simulink model "Dinamica_Residual"  (R2023b)
settings: Solver=VariableStepAuto  StartTime=0.0  StopTime=10.0  RelTol=1e-3
values from neighbouring files (symbols this model uses):
  lambda_m = 0.016    [parametros_proyecto2.m]
  Ld = 6.6e-3    (= 0.0066)    [parametros_proyecto2.m]
  Lls = 0.8e-3    (= 0.0008)    [parametros_proyecto2.m]
  Lq = 5.8e-3    (= 0.0058)    [parametros_proyecto2.m]
  r = 120    [parametros_proyecto2.m]
  Rs_ref = 1.02    [parametros_proyecto2.m]
  Rts_amb = 146.7    [parametros_proyecto2.m]
undefined symbols (not defined in the file or in its folder): b_eq, cts, J_eq, P_p, R_s
settings Model: Creator=ignab  LastModifiedBy=ignab

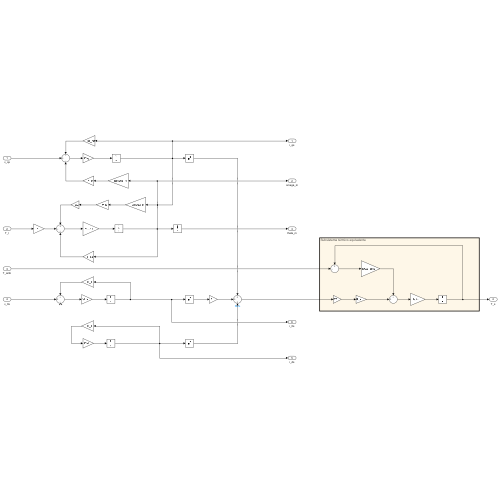
[thumbnail: Simulink's stored preview of the top-level diagram]
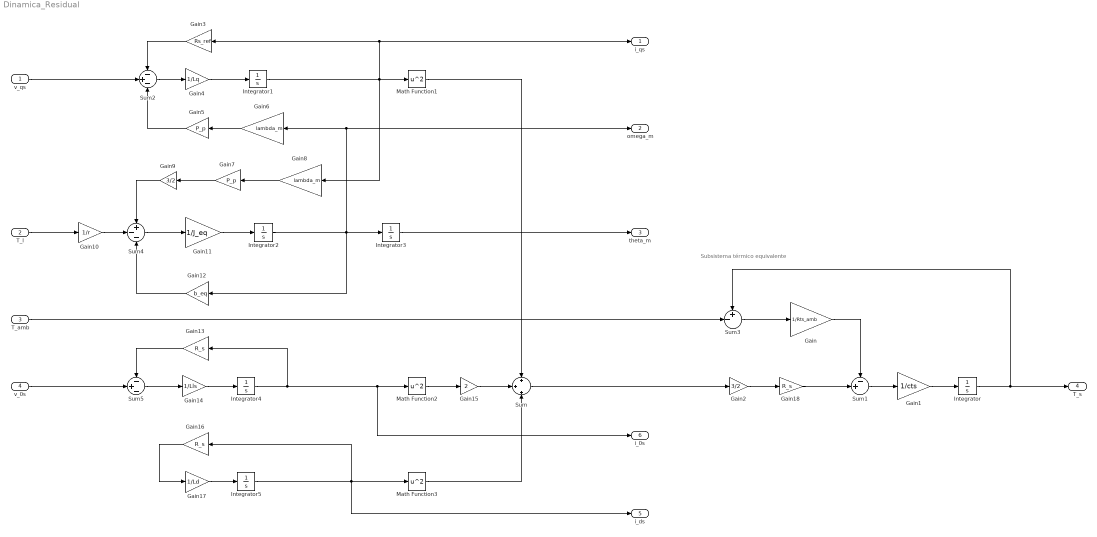
== system Dinamica_Residual ==
  note: Subsistema térmico equivalente
  v_qs : Inport
  T_l : Inport  Port=2
  T_amb : Inport  Port=3
  v_0s : Inport  Port=4
  Gain : Gain  Gain=1/Rts_amb
  Gain1 : Gain  Gain=1/cts
  Gain10 : Gain  Gain=1/r
  Gain11 : Gain  Gain=1/J_eq
  Gain12 : Gain  Gain=b_eq
  Gain13 : Gain  Gain=R_s
  Gain14 : Gain  Gain=1/Lls
  Gain15 : Gain  Gain=2
  Gain16 : Gain  Gain=R_s
  Gain17 : Gain  Gain=1/Ld
  Gain18 : Gain  Gain=R_s
  Gain2 : Gain  Gain=3/2
  Gain3 : Gain  Gain=Rs_ref
  Gain4 : Gain  Gain=1/Lq
  Gain5 : Gain  Gain=P_p
  Gain6 : Gain  Gain=lambda_m
  Gain7 : Gain  Gain=P_p
  Gain8 : Gain  Gain=lambda_m
  Gain9 : Gain  Gain=3/2
  Integrator{,1..5} (6 alike) : Integrator
  Math Function1 : Math  Operator=square
  Math Function2 : Math  Operator=square
  Math Function3 : Math  Operator=square
  Sum : Sum  Inputs=+|+|+
  Sum1 : Sum  Inputs=-+|
  Sum2 : Sum  Inputs=-+-
  Sum3 : Sum  Inputs=+-|
  Sum4 : Sum  Inputs=+--
  Sum5 : Sum  Inputs=-+-
  i_qs : Outport
  omega_m : Outport  Port=2
  theta_m : Outport  Port=3
  T_s : Outport  Port=4
  i_ds : Outport  Port=5
  i_0s : Outport  Port=6
  wires:
  T_amb/1 -> Sum3/2
  Sum3/1 -> Gain/1
  Gain/1 -> Sum1/1
  Sum1/1 -> Gain1/1
  Gain1/1 -> Integrator/1
  Integrator/1 -> T_s/1, Sum3/1
  v_qs/1 -> Sum2/2
  Gain5/1 -> Sum2/3
  Gain3/1 -> Sum2/1
  Sum2/1 -> Gain4/1
  Gain4/1 -> Integrator1/1
  Gain6/1 -> Gain5/1
  Integrator1/1 -> Gain3/1, i_qs/1, Math Function1/1, Gain8/1
  Gain8/1 -> Gain7/1
  Gain7/1 -> Gain9/1
  Gain9/1 -> Sum4/1
  Gain12/1 -> Sum4/3
  Sum4/1 -> Gain11/1
  Gain11/1 -> Integrator2/1
  Integrator2/1 -> Integrator3/1, Gain12/1, omega_m/1, Gain6/1
  Gain10/1 -> Sum4/2
  T_l/1 -> Gain10/1
  Integrator4/1 -> i_0s/1, Math Function2/1, Gain13/1
  v_0s/1 -> Sum5/2
  Sum5/1 -> Gain14/1
  Gain14/1 -> Integrator4/1
  Gain13/1 -> Sum5/1
  Gain17/1 -> Integrator5/1
  Gain16/1 -> Gain17/1
  Integrator5/1 -> Gain16/1, Math Function3/1, i_ds/1
  Math Function2/1 -> Gain15/1
  Gain15/1 -> Sum/2
  Math Function1/1 -> Sum/1
  Math Function3/1 -> Sum/3
  Sum/1 -> Gain2/1
  Gain2/1 -> Gain18/1
  Gain18/1 -> Sum1/2
  Integrator3/1 -> theta_m/1
